simulink model "simple_HGO_ASMC"  (R2023a)
settings: Solver=ode1  StartTime=0.0  StopTime=60  FixedStep=0.01  RelTol=1e-3
libraries: robotcorelib x1
settings Model: Creator=Adan Daniel  LastModifiedBy=Adan Daniel
settings OptimizationCC: ReuseModelBlockBuffer=off

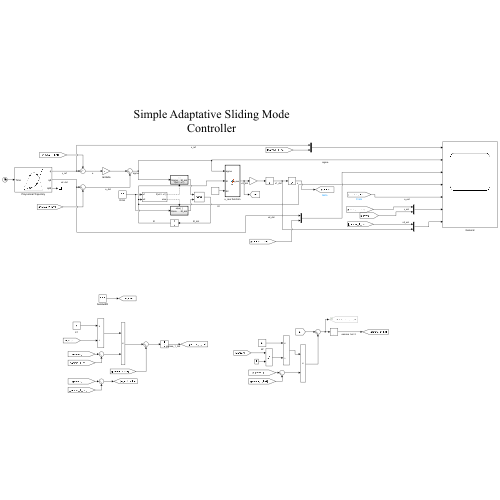
[thumbnail: Simulink's stored preview of the top-level diagram]
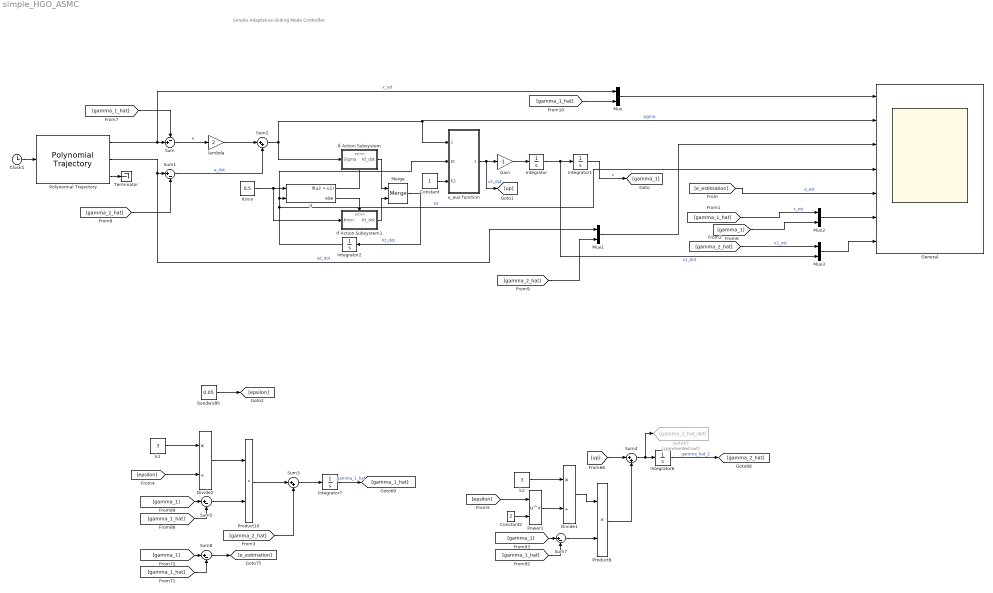
== system simple_HGO_ASMC ==
  note: Simple Adaptative Sliding Mode Controller
  Clock1 : Clock
  Constant : Constant
  Constant2 : Constant  Value=2
  Divide1 : Product  Inputs=*/
  Divide2 : Product  Inputs=*/
  Gain : Gain  Gain=-1
  General : Scope  NumInputPorts=7
  Goto67 : Goto  Commented=on  GotoTag=gamma_2_hat_dot
  If : If  NumInputs=2  IfExpression=u2 > u1
  If Action Subsystem : Subsystem  TreatAsAtomicUnit=on
  If Action Subsystem1 : Subsystem  TreatAsAtomicUnit=on
  Integrator{,1..2,6..7} (5 alike) : Integrator
  Kmin : Constant  Value=0.5
  Merge : Merge
  Mux{,1..3} (4 alike) : Mux  Inputs=2
  Polynomial Trajectory : robotcorelib/Polynomial Trajectory  WaypointSource=Internal  Waypoints=[1, 2, 0, -2, 0, 1]  TimePoints=[0, 12, 24, 36, 48, 60]  TimeInterval=[ 1, 4 ]  Method=Cubic Polynomial  ParameterSource=Internal  VelocityBoundaryCondition=zeros( 1, 6 )  AccelerationBoundaryCondition=zeros( 2, 5 )  SimulateUsing=Interpreted execution
  Power1 : Math  Operator=pow
  Product10 : Product
  Product8 : Product
  Sum : Sum  Inputs=-+|
  Sum{1,5,7..8} (4 alike) : Sum  Inputs=|+-
  Sum2 : Sum  Inputs=|++
  Sum3 : Sum  Inputs=|++
  Sum4 : Sum  Inputs=|++
  Terminator : Terminator
  bandwidth : Constant  Value=0.05
  k1 : Constant  Value=3
  k2 : Constant  Value=3
  lambda : Gain  Gain=2
  u_aux function : MATLAB Function  TreatAsAtomicUnit=on
  wires:
  Mux1/1 -> General/3
  Integrator1/1 -> [gamma_1]  "x"
  Integrator/1 -> Mux3/2, Integrator1/1  "x1_dot"
  Sum/1 -> lambda/1  "e"
  Sum1/1 -> Sum2/2  "e_dot"
  Sum2/1 -> If Action Subsystem/1(Sigma), u_aux function/1(sigma), General/2  "sigma"
  Mux/1 -> General/1
  lambda/1 -> Sum2/1
  u_aux function/1(u_aux) -> [up], Gain/1  "x2_dot"
  Merge/1 -> Integrator2/1  "Kt_dot"
  Integrator2/1 -> u_aux function/2(Kt), If/2, General/4  "Kt"
  Kmin/1 -> If/1, If Action Subsystem1/1(Kmin)
  If/1 -> If Action Subsystem/Action
  If/2 -> If Action Subsystem1/Action
  If Action Subsystem/1(Kt_dot) -> Merge/1
  If Action Subsystem1/1(Kt_dot) -> Merge/2
  Constant/1 -> u_aux function/3(K2)
  Gain/1 -> Integrator/1
  Polynomial Trajectory/1 -> Mux/1, Sum/2  "x_ref"
  Polynomial Trajectory/2 -> Mux1/1, Sum1/1  "xd_dot"
  Clock1/1 -> Polynomial Trajectory/1
  Polynomial Trajectory/3 -> Terminator/1
  Sum5/1 -> Product10/2
  Sum3/1 -> Integrator7/1
  [gamma_1_hat] -> Sum5/2
  k1/1 -> Divide2/1
  Product10/1 -> Sum3/1
  Integrator7/1 -> [gamma_1_hat]  "gamma_1_hat"
  [epsilon] -> Divide2/2
  [gamma_1] -> Sum5/1
  Divide2/1 -> Product10/1
  [gamma_2_hat] -> Sum3/2
  [gamma_1_hat] -> Sum7/2
  [gamma_1] -> Sum7/1
  Constant2/1 -> Power1/2
  [epsilon] -> Power1/1
  [gamma_1] -> Sum8/1
  Sum7/1 -> Product8/2
  Power1/1 -> Divide1/2
  [gamma_1_hat] -> Sum8/2
  Sum8/1 -> [e_estimation]
  k2/1 -> Divide1/1
  Integrator6/1 -> [gamma_2_hat]  "gamma_hat_2"
  Divide1/1 -> Product8/1
  Sum4/1 -> Goto67/1, Integrator6/1
  [up] -> Sum4/1
  Product8/1 -> Sum4/2
  [e_estimation] -> General/5  "e_est"
  [gamma_1_hat] -> Mux2/1  "x_est"
  [gamma_2_hat] -> Mux3/1  "x2_est"
  bandwidth/1 -> [epsilon]
  Mux2/1 -> General/6
  [gamma_1] -> Mux2/2
  Mux3/1 -> General/7
  [gamma_1_hat] -> Sum/1
  [gamma_2_hat] -> Sum1/2
  [gamma_2_hat] -> Mux1/2
  [gamma_1_hat] -> Mux/2

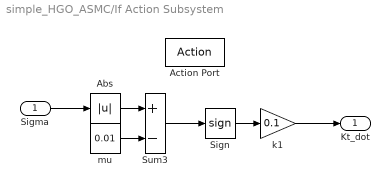
== system simple_HGO_ASMC/If Action Subsystem ==
  Sigma : Inport
  Action Port : ActionPort  ActionPortLabel=if(u2 > u1)
  Abs : Abs  SaturateOnIntegerOverflow=off
  Sign : Signum
  Sum3 : Sum  Inputs=+-
  k1 : Gain  Gain=0.1
  mu : Constant  Value=0.01
  Kt_dot : Outport
  wires:
  Sign/1 -> k1/1
  mu/1 -> Sum3/2
  Sum3/1 -> Sign/1
  Abs/1 -> Sum3/1
  k1/1 -> Kt_dot/1
  Sigma/1 -> Abs/1

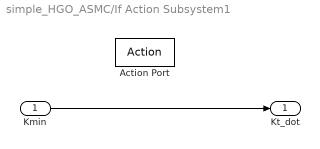
== system simple_HGO_ASMC/If Action Subsystem1 ==
  Kmin : Inport
  Action Port : ActionPort  ActionPortLabel=else
  Kt_dot : Outport
  wires:
  Kmin/1 -> Kt_dot/1

== matlab function simple_HGO_ASMC/u_aux function ==
  data: sigma input; u_aux output; Kt input; K2 input
function u_aux = fcn(sigma, Kt, K2)

u_aux = - Kt * (abs(sigma) ^ (0.5)) * sign(sigma) - K2 * sigma;
